simulink model "LUP_export_in_simulink"  (R2023a)
settings: Solver=VariableStepAuto  StartTime=0.0  StopTime=10.0  RelTol=1e-3
model workspace (MAT data in the model file):
  surfaceBlockParameters = Simulink.LookupTable
  surfaceBlockParameters.Table = Simulink.lookuptable.Table
  surfaceBlockParameters.Table.Value = [0.3  0.25  0.25  0.25  0.25  0.25  0.25  0.25  0.25  0.25; 0.318655287955  0.276524695618  0.25  0.25  0.25  0.25  0.25  0.25  0.25  0.25; 0.362852349848  0.313586462738  0.282466191975  0.25  0.25  0.25  0.25  0.25  0.25  0.25; 0.476014258567  0.368194700949  0.324320626752  0.289627337745  0.25  0.25  0.25  0.25  0.25  0.25; 0.545722661004  0.442668923785  0.366317292779  0.342629293191  0.296813123056  0.25  0.25  0.25  0.25  0.25; 0.527120631842  0.515194727142  0.42660589383  0.370557593233  0.360706092628  0.304063210196  0.25  0.25  0.25  0.25; 0.536676995908  0.508164349971  0.463570071436  0.413712707012  0.390959342679  0.365951297778  0.311320122877  0.25  0.25  0.25; 0.536631925819  0.485318874986  0.439465117375  0.419913246351  0.412168854759  0.409242969026  0.371196502928  0.318577035558  0.25  0.25; 0.49698991044  0.463570071436  0.428653626497  0.418274281378  0.415124927195  0.418368561131  0.400902176424  0.376441708078  0.326579084412  0.366890238521; 0.479550409548  0.44163978814  0.418488047816  0.412168854759  0.418286941457  0.425759580228  0.40949768382  0.391587570223  0.374869743926  0.359080208923; 0.463570071436  0.428653626497  0.418488047816  0.416214093589  0.418733336557  0.425759580228  0.395110735508  0.379052188577  0.365842695466  0.351156577055]
  surfaceBlockParameters.Table.Dimensions = [11 10]
  surfaceBlockParameters.Table.DataType = 'auto'
  surfaceBlockParameters.Table.FieldName = 'Table_efficiency'
  surfaceBlockParameters.Breakpoints(1) = Simulink.lookuptable.Breakpoint
  surfaceBlockParameters.Breakpoints(1).Value = [3700 4500 5300 6100 6900 7700 8500 9300 10100 10900 11700]
  surfaceBlockParameters.Breakpoints(1).TunableSizeName = 'N1'
  surfaceBlockParameters.Breakpoints(1).Dimensions = [1 11]
  surfaceBlockParameters.Breakpoints(1).DataType = 'auto'
  surfaceBlockParameters.Breakpoints(1).FieldName = 'BP1_NTurbine'
  surfaceBlockParameters.Breakpoints(2) = Simulink.lookuptable.Breakpoint
  surfaceBlockParameters.Breakpoints(2).Value = [5.7 38.7 71.7 104.7 137.7 170.7 203.7 236.7 269.7 302.7]
  surfaceBlockParameters.Breakpoints(2).TunableSizeName = 'N2'
  surfaceBlockParameters.Breakpoints(2).Dimensions = [1 10]
  surfaceBlockParameters.Breakpoints(2).DataType = 'auto'
  surfaceBlockParameters.Breakpoints(2).FieldName = 'BP2_PFuel'
  surfaceBlockParameters.AllowMultipleInstancesOfTypeToHaveDifferentTableBreakpointSizes = 0
  surfaceBlockParameters.SupportTunableSize = 0
  surfaceBlockParameters.StructTypeInfo = Simulink.lookuptable.StructTypeInfo
  surfaceBlockParameters.StructTypeInfo.Name = 'surfaceBlockParameters_type'
  surfaceBlockParameters.StructTypeInfo.DataScope = 'Auto'
settings Model: Creator=kroblet  LastModifiedBy=kroblet

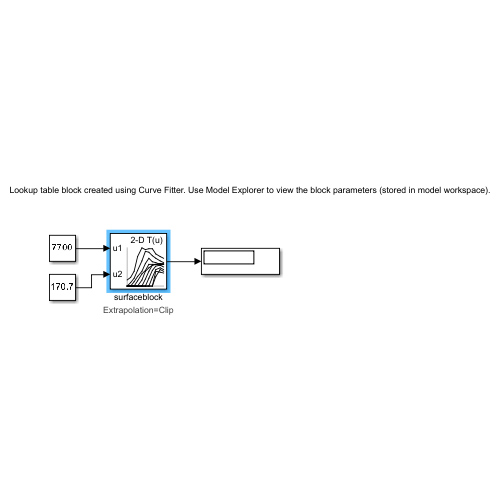
[thumbnail: Simulink's stored preview of the top-level diagram]
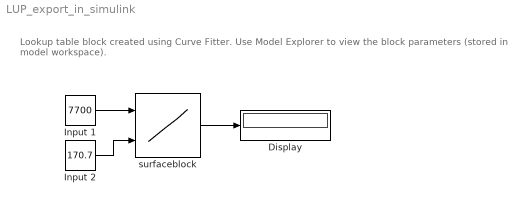
== system LUP_export_in_simulink ==
  note: Lookup table block created using Curve Fitter. Use Model Explorer to view the block parameters (stored in model workspace).
  Display : Display
  Input 1 : Constant  Value=7700
  Input 2 : Constant  Value=170.7
  surfaceblock : Lookup_n-D  DataSpecification=Lookup table object  LookupTableObject=surfaceBlockParameters  BreakpointsForDimension1=[1:3]  BreakpointsForDimension2=[1:3]  ExtrapMethod=Clip  InternalRulePriority=Speed  RndMeth=Simplest
      settings: AttributesFormatString=Extrapolation=%<ExtrapMethod>  InputPortMap=u0,u1
  wires:
  Input 1/1 -> surfaceblock/1
  Input 2/1 -> surfaceblock/2
  surfaceblock/1 -> Display/1
